simulink model "untitled1"  (R2020b)
settings: Solver=VariableStepAuto  StartTime=0.0  StopTime=10.0  RelTol=1e-3
settings Model: Creator=Hp  LastModifiedBy=Hp

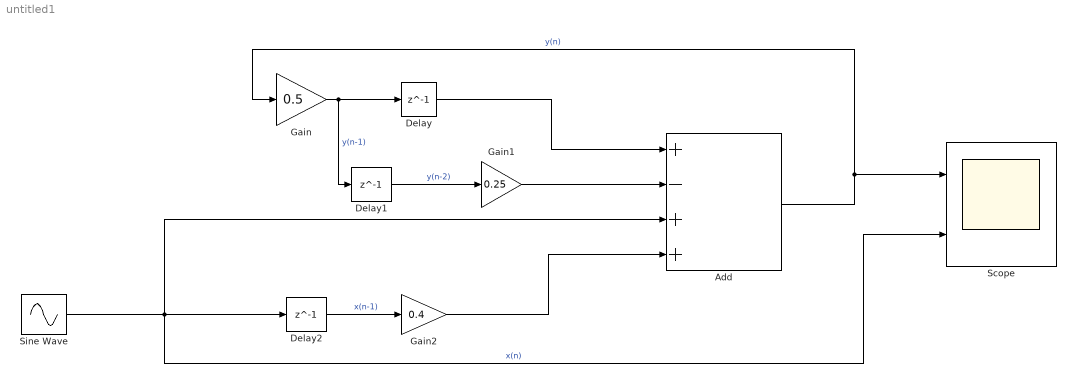
== system untitled1 ==
  Add : Sum  Inputs=+-++
  Delay : Delay  DelayLength=1
  Delay1 : Delay  DelayLength=1
  Delay2 : Delay  DelayLength=1
  Gain : Gain  Gain=0.5
  Gain1 : Gain  Gain=0.25
  Gain2 : Gain  Gain=0.4
  Scope : Scope  NumInputPorts=2
  Sine Wave : Sin  SampleTime=0
  wires:
  Gain/1 -> Delay1/1, Delay/1  "y(n-1)"
  Delay/1 -> Add/1
  Add/1 -> Gain/1, Scope/1  "y(n)"
  Sine Wave/1 -> Delay2/1, Add/3, Scope/2  "x(n)"
  Delay2/1 -> Gain2/1  "x(n-1)"
  Gain2/1 -> Add/4
  Delay1/1 -> Gain1/1  "y(n-2)"
  Gain1/1 -> Add/2
